simulink model "ELQR_P_Controller"  (R2020b)
settings: Solver=VariableStepAuto  StartTime=0.0  StopTime=70  MaxStep=0.01  RelTol=1e-3
values from neighbouring files (symbols this model uses):
  A_real = [0 0 0 1 0 0 0 0 0 0 0 0 ... (first row only)    [LQG_calcs.m]
  B_real = [0 0 0 0 ... (first row only)    [LQG_calcs.m]
  C_real = eye(12)    [LQG_calcs.m]
  D_real = B_real    [LQG_calcs.m]
  Del = [0 0.025 1]    [LQG_calcs.m]
  g = 9.8066    [LQG_calcs.m]
  m = 0.915    [LQG_calcs.m]
undefined symbols (not defined in the file or in its folder): K
libraries: pid_lib x3, sharedtransform x1, uavutilslib x1
settings Model: EnablePacing=on  Creator=tesla  LastModifiedBy=tesla
settings SolverCC: ZeroCrossAlgorithm=Adaptive  AlgebraicLoopSolver=LineSearch
settings DebuggingCC: IgnoredZcDiagnostic=none

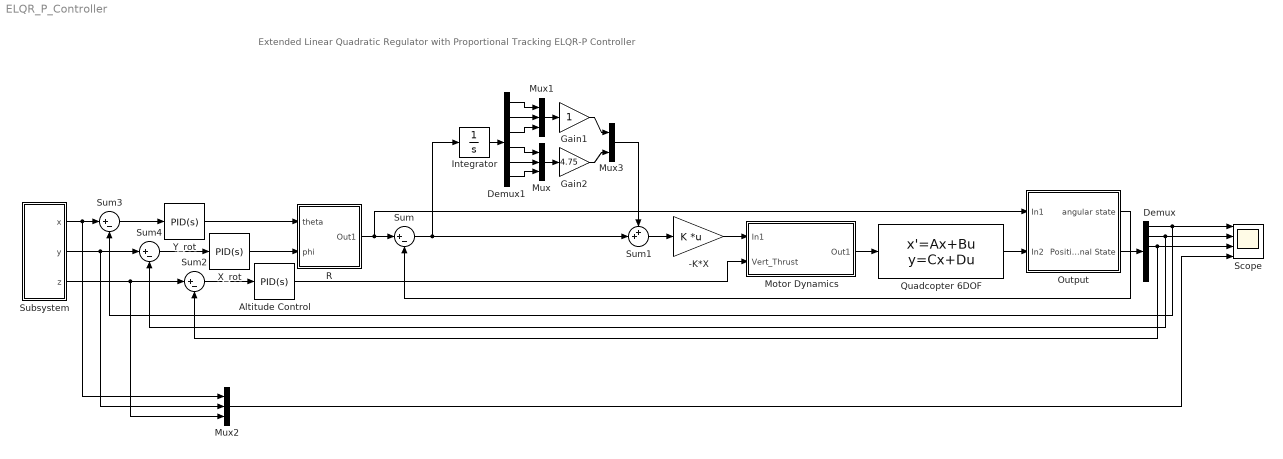
== system ELQR_P_Controller ==
  note: Extended Linear Quadratic Regulator with Proportional Tracking
      | ELQR-P Controller
  -K*X : Gain  Gain=K  Multiplication=Matrix(K*u) (u vector)
  Altitude Control : pid_lib/PID Controller  Controller=PID  Form=Parallel  TimeDomain=Continuous-time  UseExternalTs=off  SampleTime=-1  IntegratorMethod=Forward Euler  FilterMethod=Forward Euler  ControllerParametersSource=internal  P=10  I=5  D=7  UseFilter=on  N=100  TunerSelectOption=Transfer Function Based (PID Tuner App)  InitialConditionSource=internal  InitialConditionForIntegrator=0  InitialConditionForFilter=0  DifferentiatorICPrevScaledInput=0  ExternalReset=none  TrackingMode=off  Kt=1  LimitOutput=on  SatLimitsSource=internal  UpperSaturationLimit=15  LowerSaturationLimit=0  LinearizeAsGain=off  AntiWindupMode=clamping  Kb=1  POutMin=[]  POutMax=[]  IOutMin=[]  IOutMax=[]  DOutMin=[]  DOutMax=[]  NOutMin=[]  NOutMax=[]  SumOutMin=[]  SumOutMax=[]  SaturationOutMin=[]  SaturationOutMax=[]  PParamMin=[]  PParamMax=[]  IParamMin=[]  IParamMax=[]  DParamMin=[]  DParamMax=[]  NParamMin=[]  NParamMax=[]  KbParamMin=[]  KbParamMax=[]  KtParamMin=[]  KtParamMax=[]  KbOutMin=[]  KbOutMax=[]  KtOutMin=[]  KtOutMax=[]  IntegratorOutMin=[]  IntegratorOutMax=[]  FilterOutMin=[]  FilterOutMax=[]  SumI1OutMin=[]  SumI1OutMax=[]  SumI2OutMin=[]  SumI2OutMax=[]  SumI3OutMin=[]  SumI3OutMax=[]  SumI4OutMin=[]  SumI4OutMax=[]  SumDOutMin=[]  SumDOutMax=[]  DifferentiatorOutMin=[]  DifferentiatorOutMax=[]  FilterDiffOutCoefMin=[]  FilterDiffOutCoefMax=[]  ReciprocalOutMin=[]  ReciprocalOutMax=[]  SumDenOutMin=[]  SumDenOutMax=[]  SumNumOutMin=[]  SumNumOutMax=[]  DivideOutMin=[]  DivideOutMax=[]  UdiffTsProdOutMin=[]  UdiffTsProdOutMax=[]  NTsProdOutMin=[]  NTsProdOutMax=[]  UintegralTsProdOutMin=[]  UintegralTsProdOutMax=[]  UngainTsProdOutMin=[]  UngainTsProdOutMax=[]  IntegratorContinuousStateAttributes=''  IntegratorStateMustResolveToSignalObject=off  IntegratorRTWStateStorageClass=Auto  FilterContinuousStateAttributes=''  FilterStateMustResolveToSignalObject=off  FilterRTWStateStorageClass=Auto  ParallelPVariant=InternalParameters  IdealPVariant=Disabled  IVariant=InternalParameters  DVariant=InternalParameters  IntegratorVariant=Continuous  SatVariant=Enabled  AWVariant=ContClampingParallel  PCopyVariant=Disabled  TRVariant=Disabled  FdbkBlocksVariant=Forward  IdealPFdbkVariant=Disabled  SatFdbkVariant=Disabled  DerivativeFilterVariant=ContFilter  NVariant=InternalParameters  NCopyVariant=Disabled  FilterICVariant=InternalICsFilter  IntegratorICVariant=InternalICs  ExternalResetVariant=Disabled  TRSumVariant=Passthrough  SumFdbkVariant=Disabled  SumVariant=Sum_PID  TsampFilterVariant=InternalTs  TsampNgainVariant=Passthrough  TsampIntegralVariant=Passthrough  ExternalSaturationOutDataTypeStr=Inherit: Same as second input
  Demux : Demux  Outputs=6
  Demux1 : Demux  Outputs=6
  Gain1 : Gain
  Gain2 : Gain  Gain=4.75
  Integrator : Integrator
  Motor Dynamics : Subsystem
  Mux : Mux  Inputs=3
  Mux1 : Mux  Inputs=3
  Mux2 : Mux  Inputs=3
  Mux3 : Mux  Inputs=2
  Output : Subsystem
  Quadcopter 6DOF : StateSpace  A=A_real  B=B_real  C=C_real  D=D_real  InitialCondition=[0 0 0 0 0 0 0 0 0 0 0 0]
  R : Subsystem
  Scope : Scope  NumInputPorts=4
  Subsystem : Subsystem
  Sum{,2..4} (4 alike) : Sum  Inputs=|+-
  Sum1 : Sum  Inputs=++|
  X_rot : pid_lib/PID Controller  Controller=PID  Form=Parallel  TimeDomain=Continuous-time  UseExternalTs=off  SampleTime=-1  IntegratorMethod=Forward Euler  FilterMethod=Forward Euler  ControllerParametersSource=internal  P=-0.085  I=0  D=-0.175  UseFilter=on  N=25  TunerSelectOption=Transfer Function Based (PID Tuner App)  InitialConditionSource=internal  InitialConditionForIntegrator=0  InitialConditionForFilter=0  DifferentiatorICPrevScaledInput=0  ExternalReset=none  TrackingMode=off  Kt=1  LimitOutput=on  SatLimitsSource=internal  UpperSaturationLimit=1  LowerSaturationLimit=-1  LinearizeAsGain=on  AntiWindupMode=clamping  Kb=1  POutMin=[]  POutMax=[]  IOutMin=[]  IOutMax=[]  DOutMin=[]  DOutMax=[]  NOutMin=[]  NOutMax=[]  SumOutMin=[]  SumOutMax=[]  SaturationOutMin=[]  SaturationOutMax=[]  PParamMin=[]  PParamMax=[]  IParamMin=[]  IParamMax=[]  DParamMin=[]  DParamMax=[]  NParamMin=[]  NParamMax=[]  KbParamMin=[]  KbParamMax=[]  KtParamMin=[]  KtParamMax=[]  KbOutMin=[]  KbOutMax=[]  KtOutMin=[]  KtOutMax=[]  IntegratorOutMin=[]  IntegratorOutMax=[]  FilterOutMin=[]  FilterOutMax=[]  SumI1OutMin=[]  SumI1OutMax=[]  SumI2OutMin=[]  SumI2OutMax=[]  SumI3OutMin=[]  SumI3OutMax=[]  SumI4OutMin=[]  SumI4OutMax=[]  SumDOutMin=[]  SumDOutMax=[]  DifferentiatorOutMin=[]  DifferentiatorOutMax=[]  FilterDiffOutCoefMin=[]  FilterDiffOutCoefMax=[]  ReciprocalOutMin=[]  ReciprocalOutMax=[]  SumDenOutMin=[]  SumDenOutMax=[]  SumNumOutMin=[]  SumNumOutMax=[]  DivideOutMin=[]  DivideOutMax=[]  UdiffTsProdOutMin=[]  UdiffTsProdOutMax=[]  NTsProdOutMin=[]  NTsProdOutMax=[]  UintegralTsProdOutMin=[]  UintegralTsProdOutMax=[]  UngainTsProdOutMin=[]  UngainTsProdOutMax=[]  IntegratorContinuousStateAttributes=''  IntegratorStateMustResolveToSignalObject=off  IntegratorRTWStateStorageClass=Auto  FilterContinuousStateAttributes=''  FilterStateMustResolveToSignalObject=off  FilterRTWStateStorageClass=Auto  ParallelPVariant=InternalParameters  IdealPVariant=Disabled  IVariant=InternalParameters  DVariant=InternalParameters  IntegratorVariant=Continuous  SatVariant=Enabled  AWVariant=ContClampingParallel  PCopyVariant=Disabled  TRVariant=Disabled  FdbkBlocksVariant=Forward  IdealPFdbkVariant=Disabled  SatFdbkVariant=Disabled  DerivativeFilterVariant=ContFilter  NVariant=InternalParameters  NCopyVariant=Disabled  FilterICVariant=InternalICsFilter  IntegratorICVariant=InternalICs  ExternalResetVariant=Disabled  TRSumVariant=Passthrough  SumFdbkVariant=Disabled  SumVariant=Sum_PID  TsampFilterVariant=InternalTs  TsampNgainVariant=Passthrough  TsampIntegralVariant=Passthrough  ExternalSaturationOutDataTypeStr=Inherit: Same as second input
  Y_rot : pid_lib/PID Controller  Controller=PID  Form=Parallel  TimeDomain=Continuous-time  UseExternalTs=off  SampleTime=-1  IntegratorMethod=Forward Euler  FilterMethod=Forward Euler  ControllerParametersSource=internal  P=0.095  I=0  D=0.175  UseFilter=on  N=25  TunerSelectOption=Transfer Function Based (PID Tuner App)  InitialConditionSource=internal  InitialConditionForIntegrator=0  InitialConditionForFilter=0  DifferentiatorICPrevScaledInput=0  ExternalReset=none  TrackingMode=off  Kt=1  LimitOutput=on  SatLimitsSource=internal  UpperSaturationLimit=1  LowerSaturationLimit=-1  LinearizeAsGain=on  AntiWindupMode=clamping  Kb=1  POutMin=[]  POutMax=[]  IOutMin=[]  IOutMax=[]  DOutMin=[]  DOutMax=[]  NOutMin=[]  NOutMax=[]  SumOutMin=[]  SumOutMax=[]  SaturationOutMin=[]  SaturationOutMax=[]  PParamMin=[]  PParamMax=[]  IParamMin=[]  IParamMax=[]  DParamMin=[]  DParamMax=[]  NParamMin=[]  NParamMax=[]  KbParamMin=[]  KbParamMax=[]  KtParamMin=[]  KtParamMax=[]  KbOutMin=[]  KbOutMax=[]  KtOutMin=[]  KtOutMax=[]  IntegratorOutMin=[]  IntegratorOutMax=[]  FilterOutMin=[]  FilterOutMax=[]  SumI1OutMin=[]  SumI1OutMax=[]  SumI2OutMin=[]  SumI2OutMax=[]  SumI3OutMin=[]  SumI3OutMax=[]  SumI4OutMin=[]  SumI4OutMax=[]  SumDOutMin=[]  SumDOutMax=[]  DifferentiatorOutMin=[]  DifferentiatorOutMax=[]  FilterDiffOutCoefMin=[]  FilterDiffOutCoefMax=[]  ReciprocalOutMin=[]  ReciprocalOutMax=[]  SumDenOutMin=[]  SumDenOutMax=[]  SumNumOutMin=[]  SumNumOutMax=[]  DivideOutMin=[]  DivideOutMax=[]  UdiffTsProdOutMin=[]  UdiffTsProdOutMax=[]  NTsProdOutMin=[]  NTsProdOutMax=[]  UintegralTsProdOutMin=[]  UintegralTsProdOutMax=[]  UngainTsProdOutMin=[]  UngainTsProdOutMax=[]  IntegratorContinuousStateAttributes=''  IntegratorStateMustResolveToSignalObject=off  IntegratorRTWStateStorageClass=Auto  FilterContinuousStateAttributes=''  FilterStateMustResolveToSignalObject=off  FilterRTWStateStorageClass=Auto  ParallelPVariant=InternalParameters  IdealPVariant=Disabled  IVariant=InternalParameters  DVariant=InternalParameters  IntegratorVariant=Continuous  SatVariant=Enabled  AWVariant=ContClampingParallel  PCopyVariant=Disabled  TRVariant=Disabled  FdbkBlocksVariant=Forward  IdealPFdbkVariant=Disabled  SatFdbkVariant=Disabled  DerivativeFilterVariant=ContFilter  NVariant=InternalParameters  NCopyVariant=Disabled  FilterICVariant=InternalICsFilter  IntegratorICVariant=InternalICs  ExternalResetVariant=Disabled  TRSumVariant=Passthrough  SumFdbkVariant=Disabled  SumVariant=Sum_PID  TsampFilterVariant=InternalTs  TsampNgainVariant=Passthrough  TsampIntegralVariant=Passthrough  ExternalSaturationOutDataTypeStr=Inherit: Same as second input
  wires:
  Sum/1 -> Integrator/1, Sum1/2
  -K*X/1 -> Motor Dynamics/1(In1)
  Sum1/1 -> -K*X/1
  Integrator/1 -> Demux1/1
  Demux1/1 -> Mux1/1
  Demux1/4 -> Mux/1
  Demux1/5 -> Mux/2
  Demux1/6 -> Mux/3
  Mux/1 -> Gain2/1
  Demux1/2 -> Mux1/2
  Demux1/3 -> Mux1/3
  Mux1/1 -> Gain1/1
  Gain1/1 -> Mux3/1
  Gain2/1 -> Mux3/2
  Mux3/1 -> Sum1/1
  Motor Dynamics/1(Out1) -> Quadcopter 6DOF/1
  Altitude Control/1 -> Motor Dynamics/2(Vert_Thrust)
  Sum2/1 -> Altitude Control/1
  R/1(Out1) -> Output/1(In1), Sum/1
  Quadcopter 6DOF/1 -> Output/2(In2)
  Output/1(angular state) -> Sum/2
  Output/2(Positional State) -> Demux/1
  Demux/3 -> Scope/3, Sum2/2
  Sum3/1 -> Y_rot/1
  Demux/1 -> Scope/1, Sum3/2
  Y_rot/1 -> R/1(theta)
  Sum4/1 -> X_rot/1
  X_rot/1 -> R/2(phi)
  Demux/2 -> Scope/2, Sum4/2
  Subsystem/1(x) -> Mux2/1, Sum3/1
  Subsystem/3(z) -> Mux2/3, Sum2/1
  Subsystem/2(y) -> Mux2/2, Sum4/1
  Mux2/1 -> Scope/4

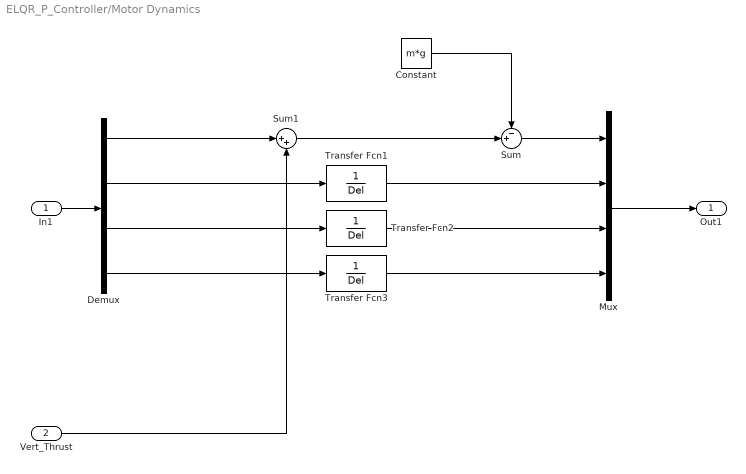
== system ELQR_P_Controller/Motor Dynamics ==
  In1 : Inport
  Vert_Thrust : Inport  Port=2
  Constant : Constant  Value=m*g
  Demux : Demux
  Mux : Mux
  Sum : Sum  Inputs=-+|
  Sum1 : Sum  Inputs=|++
  Transfer Fcn1 : TransferFcn  Denominator=Del
  Transfer Fcn2 : TransferFcn  Denominator=Del
  Transfer Fcn3 : TransferFcn  Denominator=Del
  Out1 : Outport
  wires:
  In1/1 -> Demux/1
  Demux/1 -> Sum1/1
  Demux/2 -> Transfer Fcn1/1
  Demux/3 -> Transfer Fcn2/1
  Demux/4 -> Transfer Fcn3/1
  Mux/1 -> Out1/1
  Transfer Fcn3/1 -> Mux/4
  Transfer Fcn2/1 -> Mux/3
  Transfer Fcn1/1 -> Mux/2
  Sum1/1 -> Sum/2
  Sum/1 -> Mux/1
  Constant/1 -> Sum/1
  Vert_Thrust/1 -> Sum1/2

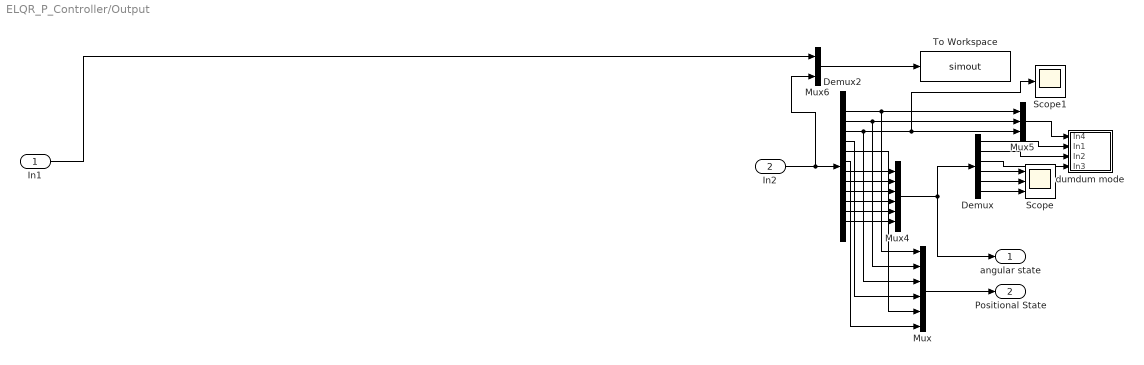
== system ELQR_P_Controller/Output ==
  In1 : Inport
  In2 : Inport  Port=2
  Demux : Demux  Outputs=6
  Demux2 : Demux  Outputs=12
  Mux : Mux  Inputs=6
  Mux4 : Mux  Inputs=6
  Mux5 : Mux  Inputs=3
  Mux6 : Mux  Inputs=2
  Scope : Scope  NumInputPorts=3
  Scope1 : Scope
  To Workspace : ToWorkspace  VariableName=simout  SaveFormat=Timeseries  SampleTime=-1
  dumdum mode : Subsystem
  angular state : Outport
  Positional State : Outport  Port=2
  wires:
  Demux2/2 -> Mux/2, Mux5/2
  Demux2/1 -> Mux/1, Mux5/1
  Demux2/7 -> Mux4/1
  Demux/2 -> dumdum mode/3(In2)
  Demux/3 -> dumdum mode/4(In3)
  Demux2/10 -> Mux4/4
  Demux/1 -> dumdum mode/2(In1)
  Demux/4 -> Scope/1
  In2/1 -> Mux6/2, Demux2/1
  Demux2/8 -> Mux4/2
  Demux/5 -> Scope/2
  Mux6/1 -> To Workspace/1
  Demux2/11 -> Mux4/5
  Mux5/1 -> dumdum mode/1(In4)
  Demux2/3 -> Mux/3, Scope1/1, Mux5/3
  In1/1 -> Mux6/1
  Demux2/12 -> Mux4/6
  Mux4/1 -> angular state/1, Demux/1
  Demux2/9 -> Mux4/3
  Demux/6 -> Scope/3
  Mux/1 -> Positional State/1
  Demux2/4 -> Mux/4
  Demux2/5 -> Mux/5
  Demux2/6 -> Mux/6

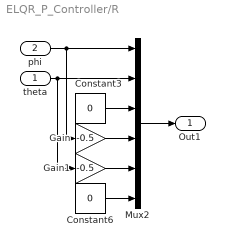
== system ELQR_P_Controller/R ==
  theta : Inport
  phi : Inport  Port=2
  Constant3 : Constant  Value=0
  Constant6 : Constant  Value=0
  Gain : Gain  Gain=-0.5
  Gain1 : Gain  Gain=-0.5
  Mux2 : Mux  Inputs=6
  Out1 : Outport
  wires:
  Mux2/1 -> Out1/1
  Constant3/1 -> Mux2/3
  phi/1 -> Mux2/1, Gain/1
  theta/1 -> Gain1/1, Mux2/2
  Constant6/1 -> Mux2/6
  Gain/1 -> Mux2/4
  Gain1/1 -> Mux2/5

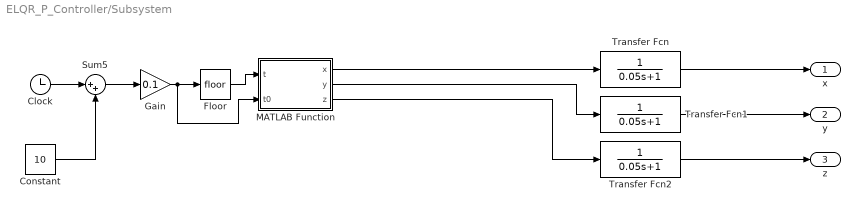
== system ELQR_P_Controller/Subsystem ==
  Clock : Clock
  Constant : Constant  Value=10
  Floor : Rounding
  Gain : Gain  Gain=0.1
  MATLAB Function : MATLAB Function  TreatAsAtomicUnit=on
  Sum5 : Sum  Inputs=|++
  Transfer Fcn : TransferFcn  Denominator=[0.05 1]
  Transfer Fcn1 : TransferFcn  Denominator=[0.05 1]
  Transfer Fcn2 : TransferFcn  Denominator=[0.05 1]
  x : Outport
  y : Outport  Port=2
  z : Outport  Port=3
  wires:
  Sum5/1 -> Gain/1
  Gain/1 -> MATLAB Function/2(t0), Floor/1
  Constant/1 -> Sum5/2
  MATLAB Function/1(x) -> Transfer Fcn/1
  MATLAB Function/3(z) -> Transfer Fcn2/1
  Clock/1 -> Sum5/1
  MATLAB Function/2(y) -> Transfer Fcn1/1
  Floor/1 -> MATLAB Function/1(t)
  Transfer Fcn/1 -> x/1
  Transfer Fcn1/1 -> y/1
  Transfer Fcn2/1 -> z/1

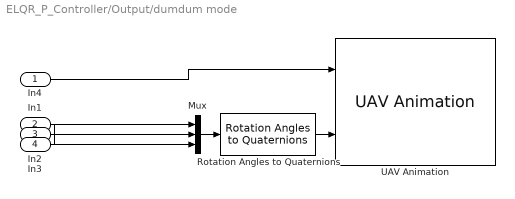
== system ELQR_P_Controller/Output/dumdum mode ==
  In4 : Inport
  In1 : Inport  Port=2
  In2 : Inport  Port=3
  In3 : Inport  Port=4
  Mux : Mux  Inputs=3
  Rotation Angles to Quaternions : sharedtransform/Rotation Angles to Quaternions  rotationOrder=ZYX  aMode=aMode
      settings: SourceProductBaseCode=AE,PW,MT,UV,VE,VP
  UAV Animation : uavutilslib/UAV Animation  UAVType=Multirotor  UAVSize=1  InertialZDirection=Up  SampleTime=-1
      settings: SourceProductBaseCode=UV
  wires:
  Rotation Angles to Quaternions/1 -> UAV Animation/2
  In1/1 -> Mux/3
  Mux/1 -> Rotation Angles to Quaternions/1
  In2/1 -> Mux/2
  In3/1 -> Mux/1
  In4/1 -> UAV Animation/1

== matlab function ELQR_P_Controller/Subsystem/MATLAB Function ==
  data: x output; t input; y output; z output; t0 input
function [x, y, z] = fcn(t,t0)

waypoints = [0 0 1
             7 0 5
             7 2 5
             2 -3 5
             -4 3 5
             5 7 5
             -3 -2 0
             -3 -2 0
             -3 -2 0
             ];
         
st = t;


x = waypoints(st,1,:)+(t0-t)*(waypoints(st+1,1,:) - waypoints(st,1,:));
y = waypoints(st,2,:)+(t0-t)*(waypoints(st+1,2,:) - waypoints(st,2,:));
z = waypoints(st,3,:)+(t0-t)*(waypoints(st+1,3,:) - waypoints(st,3,:));
